simulink model "step_input_Q3"  (R2023a)
settings: Solver=VariableStepAuto  StartTime=0.0  StopTime=10.0  RelTol=1e-3
settings Model: Creator=anshu  LastModifiedBy=anshu

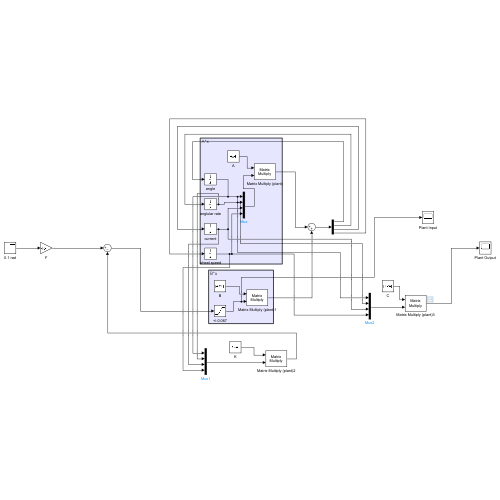
[thumbnail: Simulink's stored preview of the top-level diagram]
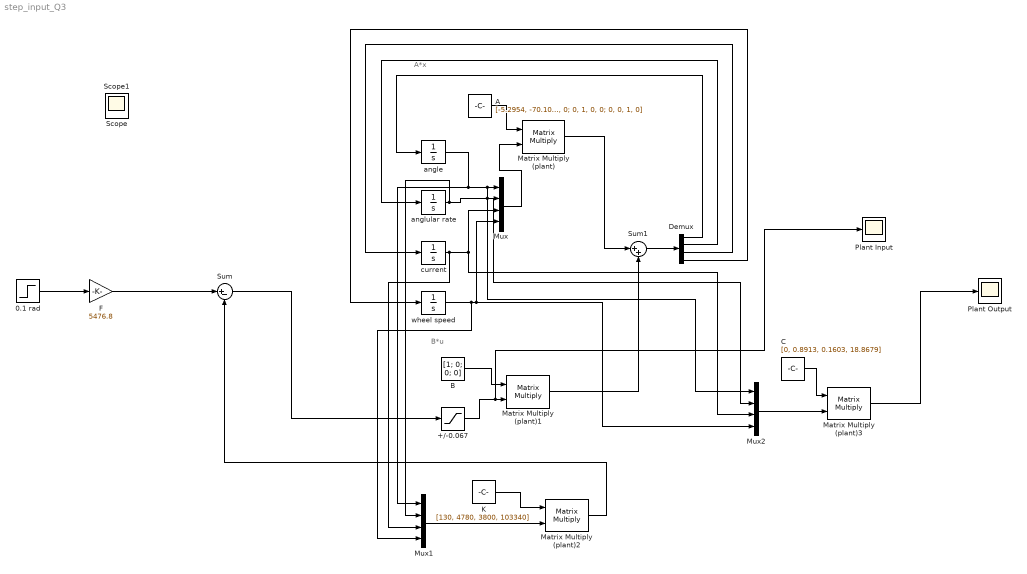
== system step_input_Q3 ==
  note: B*u
  note: A*x
  +/-0.067 : Saturate  UpperLimit=67e-3  LowerLimit=-67e-3
  0.1 rad : Step  After=0.1  SampleTime=0
  A : Constant  Value=[-5.2954, -70.1022, -343.1258, 0; 1, 0, 0, 0; 0, 1, 0, 0; 0, 0, 1, 0]
  B : Constant  Value=[1; 0; 0; 0]
  C : Constant  Value=[0, 0.8913, 0.1603, 18.8679]
  Demux : Demux
  F : Gain  Gain=5476.8
  K : Constant  Value=[130, 4780, 3800, 103340]
  Matrix Multiply (plant){,1..3} (4 alike) : Product  Multiplication=Matrix(*)
  Mux : Mux
  Mux1 : Mux
  Mux2 : Mux
  Plant Input : Scope
  Plant Output : Scope
  Sum : Sum  Inputs=|+-
  Sum1 : Sum  Inputs=|++
  angle : Integrator
  anglular rate : Integrator
  current : Integrator
  wheel speed : Integrator
  Scope : Scope
  Scope1 : Scope
  wires:
  0.1 rad/1 -> F/1
  F/1 -> Sum/1
  Matrix Multiply (plant)/1 -> Sum1/1
  Matrix Multiply (plant)1/1 -> Sum1/2
  Sum1/1 -> Demux/1
  Demux/2 -> anglular rate/1
  Demux/1 -> angle/1
  Demux/4 -> wheel speed/1
  anglular rate/1 -> Mux1/2, Mux2/2, Mux/2
  A/1 -> Matrix Multiply (plant)/1
  Mux/1 -> Matrix Multiply (plant)/2
  current/1 -> Mux1/3, Mux2/3, Mux/3
  angle/1 -> Mux/1, Mux2/1, Mux1/1
  wheel speed/1 -> Mux1/4, Mux2/4, Mux/4
  Demux/3 -> current/1
  Sum/1 -> +/-0.067/1
  +/-0.067/1 -> Plant Input/1, Matrix Multiply (plant)1/2
  B/1 -> Matrix Multiply (plant)1/1
  Mux1/1 -> Matrix Multiply (plant)2/2
  K/1 -> Matrix Multiply (plant)2/1
  Matrix Multiply (plant)2/1 -> Sum/2
  Mux2/1 -> Matrix Multiply (plant)3/2
  C/1 -> Matrix Multiply (plant)3/1
  Matrix Multiply (plant)3/1 -> Plant Output/1
